simulink subsystem "observador_estado_orden_reducido"  (R2023b)
settings: Solver=VariableStepAuto  StartTime=0.0  StopTime=10.0  RelTol=1e-3
values from neighbouring files (symbols this model uses):
  J_eq = 1.9785e-5    (= 1.9785e-05)    [diagrama_polos_y_ceros_LTI.m]    (also in main.m = 1.97847222222e-05; parametros.m = 1.97847222222e-05)
  ke_theta = 6400    [parametros.m]
  ke_w = 10240000    [parametros.m]
settings Model: Creator=nicol  LastModifiedBy=nicol

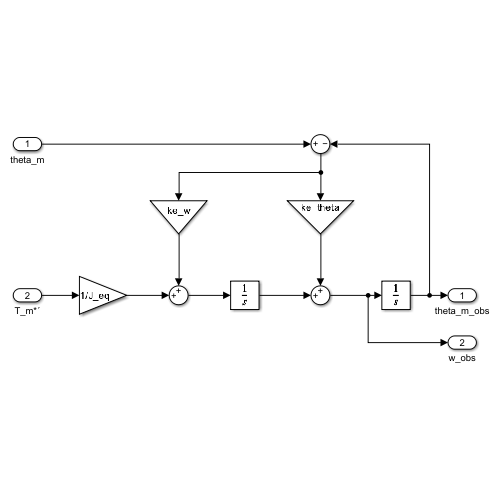
[thumbnail: Simulink's stored preview of the top-level diagram]
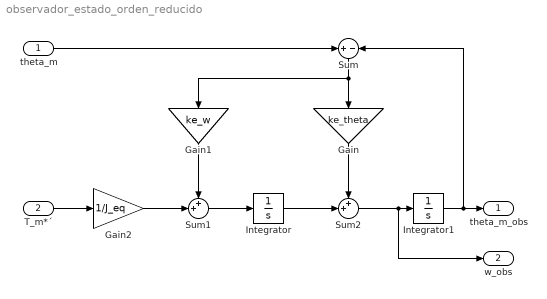
== system observador_estado_orden_reducido ==
  theta_m : Inport
  T_m*´ : Inport  Port=2
  Gain : Gain  Gain=ke_theta
  Gain1 : Gain  Gain=ke_w
  Gain2 : Gain  Gain=1/J_eq
  Integrator : Integrator
  Integrator1 : Integrator
  Sum : Sum  Inputs=+-
  Sum1 : Sum  Inputs=++|
  Sum2 : Sum  Inputs=++|
  theta_m_obs : Outport
  w_obs : Outport  Port=2
  wires:
  theta_m/1 -> Sum/1
  Sum/1 -> Gain1/1, Gain/1
  T_m*´/1 -> Gain2/1
  Gain2/1 -> Sum1/2
  Gain1/1 -> Sum1/1
  Sum1/1 -> Integrator/1
  Integrator/1 -> Sum2/2
  Gain/1 -> Sum2/1
  Sum2/1 -> w_obs/1, Integrator1/1
  Integrator1/1 -> Sum/2, theta_m_obs/1
